simulink model "FinalIteration"  (R2021b)
settings: Solver=VariableStepAuto  StartTime=0.0  StopTime=10.0  RelTol=1e-3
values from neighbouring files (symbols this model uses):
  Ball_P = 2*m*g*d*R^2/(L*(m*R^2+J))    (= 0.711925714286)    [Project.m]
  den = [1 0 0]    [Project.m]
  Kd = 2*z*Wn/Ball_P    [Project.m]
  Kp = Wn^2/Ball_P    [Project.m]
undefined symbols (not defined in the file or in its folder): xposition, yposition
settings Model: Creator=andre  LastModifiedBy=andre

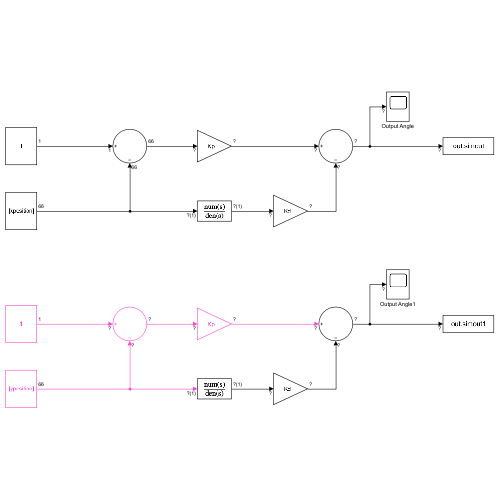
[thumbnail: Simulink's stored preview of the top-level diagram]
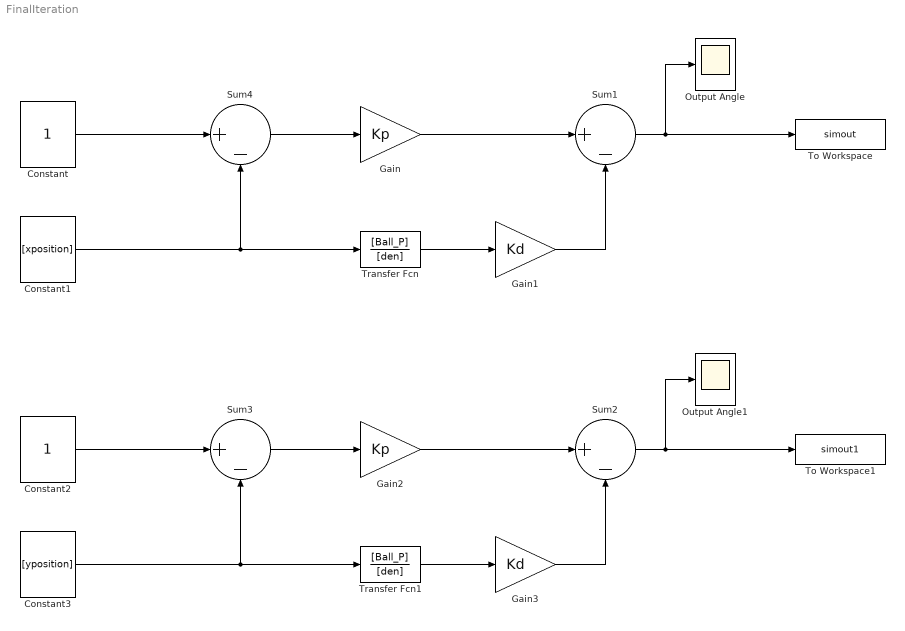
== system FinalIteration ==
  Constant : Constant
  Constant1 : Constant  Value=[xposition]
  Constant2 : Constant
  Constant3 : Constant  Value=[yposition]
  Gain : Gain  Gain=Kp  OutDataTypeStr=Inherit: Same as input
  Gain1 : Gain  Gain=Kd
  Gain2 : Gain  Gain=Kp  OutDataTypeStr=Inherit: Same as input
  Gain3 : Gain  Gain=Kd
  Output Angle : Scope
  Output Angle1 : Scope
  Sum{1..4} (4 alike) : Sum  Inputs=|+-
  To Workspace : ToWorkspace  VariableName=simout  SaveFormat=Timeseries  SampleTime=-1
  To Workspace1 : ToWorkspace  VariableName=simout1  SaveFormat=Timeseries  SampleTime=-1
  Transfer Fcn : TransferFcn  Numerator=[Ball_P]  Denominator=[den]
  Transfer Fcn1 : TransferFcn  Numerator=[Ball_P]  Denominator=[den]
  wires:
  Constant/1 -> Sum4/1
  Constant1/1 -> Transfer Fcn/1, Sum4/2
  Sum4/1 -> Gain/1
  Gain/1 -> Sum1/1
  Transfer Fcn/1 -> Gain1/1
  Gain1/1 -> Sum1/2
  Sum1/1 -> To Workspace/1, Output Angle/1
  Gain2/1 -> Sum2/1
  Gain3/1 -> Sum2/2
  Transfer Fcn1/1 -> Gain3/1
  Constant3/1 -> Transfer Fcn1/1, Sum3/2
  Constant2/1 -> Sum3/1
  Sum3/1 -> Gain2/1
  Sum2/1 -> To Workspace1/1, Output Angle1/1
